simulink model "controle_adap"  (R2020b)
settings: Solver=VariableStepAuto  StartTime=0.0  StopTime=72  RelTol=1e-3
values from neighbouring files (symbols this model uses):
  alpha = 1    [controle_adap_script.m]
  am = -1    [controle_adap_script.m]
  ap = 1    [controle_adap_script.m]
  beta = 1    [controle_adap_script.m]
  bm = 1    [controle_adap_script.m]
  bp = 1    [controle_adap_script.m]
  ref_pulse_T = 18    [controle_adap_script.m]
  ref_sin_freq = 1/ref_pulse_T    (= 0.0555555555556)    [controle_adap_script.m]
  switch_ref = 1    [controle_adap_script.m]
settings Model: Creator=lucas  LastModifiedBy=lucas

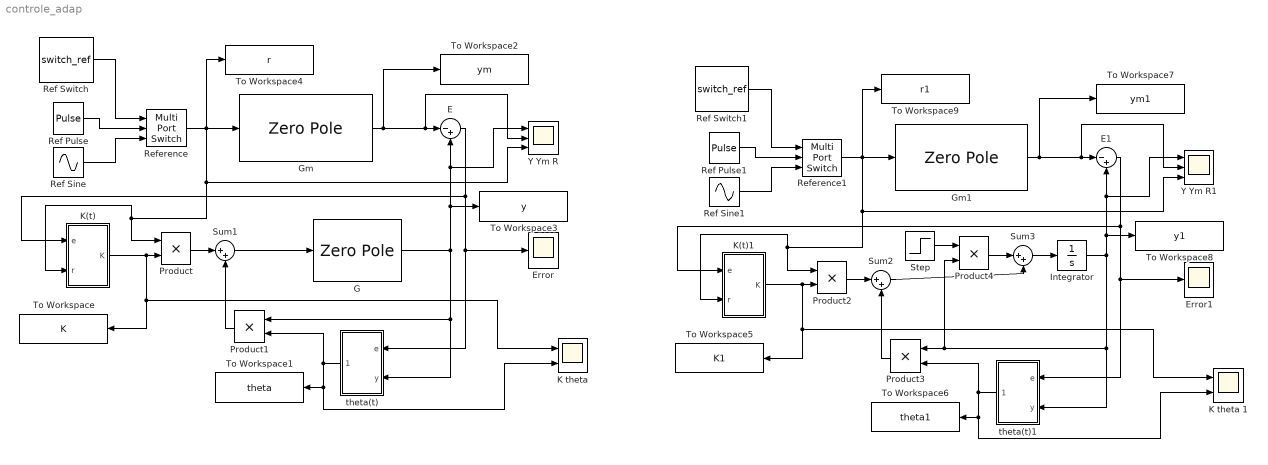
== system controle_adap ==
  E : Sum  Inputs=|-+
  E1 : Sum  Inputs=|-+
  Error : Scope
  Error1 : Scope
  G : ZeroPole  Zeros=[]  Poles=[ap]  Gain=bp
  Gm : ZeroPole  Zeros=[]  Poles=[am]  Gain=bm
  Gm1 : ZeroPole  Zeros=[]  Poles=[am]  Gain=bm
  Integrator : Integrator
  "K theta " : Scope  NumInputPorts=2
  K theta 1 : Scope  NumInputPorts=2
  K(t) : Subsystem
  K(t)1 : Subsystem
  Product{,1..4} (5 alike) : Product
  Ref Pulse : DiscretePulseGenerator  PulseType=Time based  Period=ref_pulse_T  PulseWidth=50
  Ref Pulse1 : DiscretePulseGenerator  PulseType=Time based  Period=ref_pulse_T  PulseWidth=50
  Ref Sine : Sin  Frequency=ref_sin_freq  SampleTime=0
  Ref Sine1 : Sin  Frequency=ref_sin_freq  SampleTime=0
  Ref Switch : Constant  Value=switch_ref
  Ref Switch1 : Constant  Value=switch_ref
  Reference : MultiPortSwitch  DataPortOrder=Zero-based contiguous  Inputs=2  zeroidx=on
  Reference1 : MultiPortSwitch  DataPortOrder=Zero-based contiguous  Inputs=2  zeroidx=on
  Step : Step  Time=50  Before=1  After=2  SampleTime=0
  Sum1 : Sum  Inputs=|++
  Sum2 : Sum  Inputs=|++
  Sum3 : Sum  Inputs=|++
  To Workspace : ToWorkspace  VariableName=K  SaveFormat=Timeseries  SampleTime=-1
  To Workspace1 : ToWorkspace  VariableName=theta  SaveFormat=Timeseries  SampleTime=-1
  To Workspace2 : ToWorkspace  VariableName=ym  SaveFormat=Timeseries  SampleTime=-1
  To Workspace3 : ToWorkspace  VariableName=y  SaveFormat=Timeseries  SampleTime=-1
  To Workspace4 : ToWorkspace  VariableName=r  SaveFormat=Timeseries  SampleTime=-1
  To Workspace5 : ToWorkspace  VariableName=K1  SaveFormat=Timeseries  SampleTime=-1
  To Workspace6 : ToWorkspace  VariableName=theta1  SaveFormat=Timeseries  SampleTime=-1
  To Workspace7 : ToWorkspace  VariableName=ym1  SaveFormat=Timeseries  SampleTime=-1
  To Workspace8 : ToWorkspace  VariableName=y1  SaveFormat=Timeseries  SampleTime=-1
  To Workspace9 : ToWorkspace  VariableName=r1  SaveFormat=Timeseries  SampleTime=-1
  Y Ym R : Scope  NumInputPorts=3
  Y Ym R1 : Scope  NumInputPorts=3
  theta(t) : Subsystem
  theta(t)1 : Subsystem
  wires:
  Ref Pulse/1 -> Reference/2
  Ref Sine/1 -> Reference/3
  Ref Switch/1 -> Reference/1
  Reference/1 -> Gm/1, To Workspace4/1, Y Ym R/3, K(t)/2(r), Product/1
  Gm/1 -> To Workspace2/1, Y Ym R/2, E/1
  G/1 -> Product1/1, theta(t)/2(y), To Workspace3/1, E/2, Y Ym R/1
  E/1 -> K(t)/1(e), theta(t)/1(e), Error/1
  K(t)/1(K) -> To Workspace/1, "K theta "/1, Product/2
  Product/1 -> Sum1/1
  theta(t)/1(theta) -> "K theta "/2, To Workspace1/1, Product1/2
  Product1/1 -> Sum1/2
  Sum1/1 -> G/1
  Ref Switch1/1 -> Reference1/1
  Ref Sine1/1 -> Reference1/3
  Integrator/1 -> Product4/2, Product3/1, theta(t)1/2(y), To Workspace8/1, E1/2, Y Ym R1/1
  Product2/1 -> Sum2/1
  Reference1/1 -> Gm1/1, To Workspace9/1, Y Ym R1/3, K(t)1/2(r), Product2/1
  E1/1 -> K(t)1/1(e), theta(t)1/1(e), Error1/1
  Product3/1 -> Sum2/2
  Ref Pulse1/1 -> Reference1/2
  K(t)1/1(K) -> To Workspace5/1, K theta 1/1, Product2/2
  theta(t)1/1(theta) -> K theta 1/2, To Workspace6/1, Product3/2
  Gm1/1 -> To Workspace7/1, Y Ym R1/2, E1/1
  Step/1 -> Product4/1
  Product4/1 -> Sum3/1
  Sum2/1 -> Sum3/2
  Sum3/1 -> Integrator/1

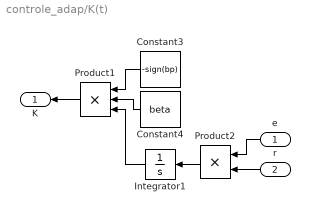
== system controle_adap/K(t) ==
  e : Inport
  r : Inport  Port=2
  Constant3 : Constant  Value=-sign(bp)
  Constant4 : Constant  Value=beta
  Integrator1 : Integrator
  Product1 : Product  Inputs=3
  Product2 : Product
  K : Outport
  wires:
  Constant3/1 -> Product1/1
  Constant4/1 -> Product1/2
  r/1 -> Product2/2
  Integrator1/1 -> Product1/3
  e/1 -> Product2/1
  Product1/1 -> K/1
  Product2/1 -> Integrator1/1

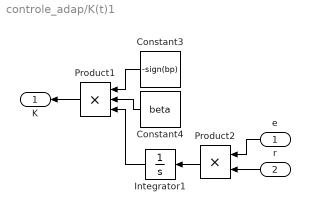
== system controle_adap/K(t)1 ==
  e : Inport
  r : Inport  Port=2
  Constant3 : Constant  Value=-sign(bp)
  Constant4 : Constant  Value=beta
  Integrator1 : Integrator
  Product1 : Product  Inputs=3
  Product2 : Product
  K : Outport
  wires:
  Constant3/1 -> Product1/1
  Constant4/1 -> Product1/2
  r/1 -> Product2/2
  Integrator1/1 -> Product1/3
  e/1 -> Product2/1
  Product1/1 -> K/1
  Product2/1 -> Integrator1/1

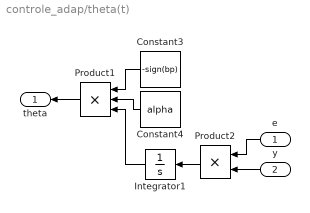
== system controle_adap/theta(t) ==
  e : Inport
  y : Inport  Port=2
  Constant3 : Constant  Value=-sign(bp)
  Constant4 : Constant  Value=alpha
  Integrator1 : Integrator
  Product1 : Product  Inputs=3
  Product2 : Product
  theta : Outport
  wires:
  Constant3/1 -> Product1/1
  Constant4/1 -> Product1/2
  y/1 -> Product2/2
  Integrator1/1 -> Product1/3
  e/1 -> Product2/1
  Product1/1 -> theta/1
  Product2/1 -> Integrator1/1

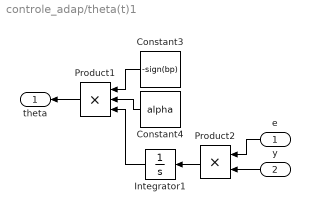
== system controle_adap/theta(t)1 ==
  e : Inport
  y : Inport  Port=2
  Constant3 : Constant  Value=-sign(bp)
  Constant4 : Constant  Value=alpha
  Integrator1 : Integrator
  Product1 : Product  Inputs=3
  Product2 : Product
  theta : Outport
  wires:
  Constant3/1 -> Product1/1
  Constant4/1 -> Product1/2
  y/1 -> Product2/2
  Integrator1/1 -> Product1/3
  e/1 -> Product2/1
  Product1/1 -> theta/1
  Product2/1 -> Integrator1/1
